simulink model "Airshow_hotpursuit_withadjustheight"  (R2012b)
settings: Solver=ode5  StartTime=0.0  StopTime=inf  FixedStep=sample_time  RelTol=1e-3
InitFcn:
  | sample_time=0.005;%0.004;%0.0025;%0.02;
  | sample_time_Vicon = 0.005;
  | DeltaT = 0.02;
  | g = 9.81;
  | H0 = g%0.3165;
  | Kl = 1;
  | 
  | Q6_mass = 0.84;
  | 
  | Q6_Omega_r = 1.5; %for horizon ref
  | Q6_Zeta_r = 0.5; %for horizon ref
  | Q6_Omega_r_h = 2;%for vertical ref
  | Q6_Zeta_r_h = 2; %for vertical ref
  | 
  | 
  | Q6_Omega = 1.5; %for horizon control
  | Q6_Zeta = 0.5; %for horizon control
  | Q6_Omega_h= 2; %for vertical control
  | Q6_Zeta_h = 0.7; %for vertical control
  | 
  | 
  | Q6_acc_max = 5;%horizontal max acc
  | Q6_acc_max_h = 3;%horizontal max acc
  | 
  | omega_circle = 72*pi/180;
  | omega_h = 0.1;%Ascending speed
  | PI = pi;
  | Circle_R = 2.5;
  | MAX_Height = -2;
undefined symbols (not defined in the file or in its folder): DiscIntNeverNeededParam
libraries: X330_Control x5, dspswit3 x5, simulink x4
(part 4 of 4)

== stateflow chart Airshow_hotpursuit_withadjustheight/UAV 1/Trajectory Logic/stateflowforwholesequence ==
  state Airborne1
    state capturing_sequence
      state caputuring_test1
        en: PosDesired = Pos; PosDesired[2] = -1.2;smooth_flag = 1;
      state capturing_sequence1
        state capturing_sequence2
          state normal_capturing1
            du: PosDesired[0] = carest[0] ; PosDesired[1] = carest[1] ; PosDesired[2] = -0.55+heightcontrol;pwm = 1650;
          state normal_capturing2
            du: PosDesired[0] = car[0] ; PosDesired[1] = car[1]; PosDesired[2] = -0.55+heightcontrol;pwm = 1250;
          state match_chk
            state caputuring_test1
              en:PosDesired = Pos;PosDesired[2] = -1.2;
            state caputuring_test2
              en: PosDesired[0] = Pos[0]+(0.25*(car[0]-Pos[0])/abs(Pos[0]-car[0]));
              PosDesired[1] = Pos[1]+0.25*(car[1]-Pos[1])/abs(Pos[1]-car[1]);
            state caputuring_test
              en: PosDesired[2] = -0.5;
            (default) -> (junction 129) : {PosDesired = Pos;pwm = 1450;PosDesired[2] = -1.2}
            (junction 129) -> Airborne1.capturing_sequence.capturing_sequence1.capturing_sequence2.match_chk.caputuring_test1 [order 1] : [abs(Pos[2]-car[2])<0.44]
            (junction 129) -> caputuring_test [order 2] : [abs(Pos[2]-car[2])>0.44]
            caputuring_test2 -> Airborne1.capturing_sequence.capturing_sequence1.capturing_sequence2.match_chk.caputuring_test1 : after(1,sec)
            caputuring_test -> caputuring_test2 : [abs(Pos[2]+0.5)<0.1]
          (default) -> normal_capturing1
          normal_capturing2 -> normal_capturing1 [order 2] : [directionflag==1]
          normal_capturing1 -> normal_capturing2 [order 2] : [(match_flag~=1)&&(directionflag~=1)]
          match_chk -> normal_capturing1 : [match_flag~=1]
          normal_capturing1 -> match_chk [order 1] : after(1,sec)
              | [match_flag==1]
          normal_capturing2 -> match_chk [order 1] : after(1,sec)
              | [match_flag==1]
        state Hover2
          en: PosDesired[2] = -1.2;
        state Hover3
          en: PosDesired[2] = -1.2;
          pwm = 1350;
        (default) -> Hover2 : {PosDesired = Pos;smooth_flag = 0;pwm = 2100;timerenable = 1;}
        Hover3 -> capturing_sequence2 : after(3,sec)
        Hover2 -> Hover3 : after(3,sec)
      state move_origin6
        du:PosDesired[1] = Pos[1];
        PosDesired[0] = (lx - PosDesired[0])*0.5*DeltaT + PosDesired[0] ;
        PosDesired[2] = -1.2;
      state move_origin5
        du:PosDesired[1] = (ly - PosDesired[1])*0.5*DeltaT + PosDesired[1] ;
        PosDesired[0] = lx;
        PosDesired[2] = -1.2;
      state hoverstate
        en:PosDesired = Pos;PosDesired[2] = -1.2;pwm = 1750;
      state hoverstate1
        en:PosDesired = Pos;PosDesired[2] = lz-0.02;pwm = 1450;
      capturing_sequence1 -> Airborne1.capturing_sequence.caputuring_test1 [order 1] : after(78,sec)
      capturing_sequence1 -> Airborne1.capturing_sequence.caputuring_test1 [order 2] : [(car[2]<-0.4)||(RC[5]<0)||(region==-1)]
      Airborne1.capturing_sequence.caputuring_test1 -> (junction 61) : [abs(Pos[2]+1.2)<0.2]
      (default) -> capturing_sequence1
      (junction 61) -> move_origin6 [order 1] : [car[2]<-0.4]
          | {pwm = 1550;}
      (junction 61) -> move_origin6 [order 2] : [(RC[5]<0)||(region==-1)||(car[2]>-0.4)]
          | {pwm = 1350;}
      move_origin6 -> move_origin5 : [(abs(lx - Pos[0]))<0.1]
      move_origin5 -> hoverstate : [(abs(lx - Pos[0])+abs(ly - Pos[1]))<0.1]
      hoverstate -> hoverstate1 : [(abs(lx - Pos[0])+abs(ly - Pos[1]))<0.1&&abs(Pos[2]+1.2)<0.15]
    state TakeOff
      du:HoverThrottle = (H0 - HoverThrottle)*2*DeltaT + HoverThrottle ;
    state Hover
      en: PosDesired[2] = -1.2;
    state move_origin
      du:PosDesired[1] = (0 - PosDesired[1])*1*DeltaT + PosDesired[1] ;PosDesired[0] = lx;
      PosDesired[2] = -1.2;
    state move_origin1
      du:PosDesired[0] = (0 - PosDesired[0])*1*DeltaT + PosDesired[0] ;PosDesired[1] = 0;
      PosDesired[2] = -1.2;
    state Hover1
      en: PosDesired[2] = -1.2;pwm = 1450;
    (default) -> TakeOff : {PosDesired = Pos;PosDesired[2] = -1.2;lx = Pos[0];ly = Pos[1];lz = Pos[2];smooth_flag = 1;pwm = 1650;timerenable = 0;}
    TakeOff -> Hover : after(3,sec)
    Hover -> move_origin : after(5,sec)
    move_origin -> move_origin1 : after(5,sec)
    move_origin1 -> Hover1 : [(abs(0 - Pos[0])+abs(0 - Pos[1]))<0.2]
        | {PosDesired = Pos;}
    Hover1 -> capturing_sequence : [RC[5] > 0]
  state Landing
    state Decsending
      en:smooth_flag = 1;pwm = 1850;
      du:PosDesired[2] = (lz - PosDesired[2])*0.05*DeltaT + PosDesired[2] ;
    state CutThrottle
      du:HoverThrottle = (0.0 - HoverThrottle)*2*DeltaT + HoverThrottle ;
    (default) -> Decsending : {PosDesired = Pos;smooth_flag = 1;}
    Decsending -> CutThrottle : [Pos[2] > lz-0.03]
  Landing -> Airborne1 : [RC[6] > 0.5]
  Airborne1 -> Landing : [RC[6] < -0.5]
  (default) -> Landing : {HoverThrottle=0.01;}
  data: PosDesired output double size=4; HoverThrottle output double size=1; RC input size=8; Pos input size=4; DeltaT parameter size=1; H0 parameter size=1; Kl parameter size=1; VelCmd local double size=2 =0; line_count local int8 size=1 =0; triangle_count local int8 size=1 =0; T_line local double size=1; omega_circle parameter size=1; PI parameter size=1; omega_h parameter; Circle_R parameter size=1; MAX_Height parameter size=1; car input size=12; carest input size=2; match_flag input; smooth_flag output boolean =0; matchx local double; matchy local double; pwm output; lx local double; ly local double; pwm1 local double; timerenable output; lz local double; laflag local boolean; directionflag input; region input; heightcontrol input

== matlab function Airshow_hotpursuit_withadjustheight/UAV 1/Vertical Controller/MATLAB Function ==
  data: u input; y output
function y = fcn(u)
%#codegen
if u > 0.5;
    y = 0;
else 
    y = 1;
end
